simulink model "simulink_test_find_K"  (R2014a)
settings: Solver=ode45  StartTime=0.0  StopTime=5000  RelTol=1e-3
values from neighbouring files (symbols this model uses):
  Gb = 200    [pole_placement.m]    (also in pole_placement2.m; time_domain.m)
  Ib = 0    [pole_placement.m]    (also in pole_placement2.m; time_domain.m)
  n = 0.142    [pole_placement.m]    (also in pole_placement2.m; time_domain.m)
  p1 = 0.035    [pole_placement.m]    (also in pole_placement2.m; time_domain.m)
  p2 = 0.05    [pole_placement.m]    (also in pole_placement2.m; time_domain.m)
  p3 = 0.000023    (= 2.3e-05)    [pole_placement.m]    (also in pole_placement2.m = 2.8e-05; time_domain.m)
  VG = 117    [pole_placement.m]    (also in pole_placement2.m; time_domain.m)
  VI = 1/0.098    (= 10.2040816327)    [pole_placement.m]    (also in pole_placement2.m; time_domain.m)
libraries: simulink x3
settings Model: Creator=joach  LastModifiedBy=joach

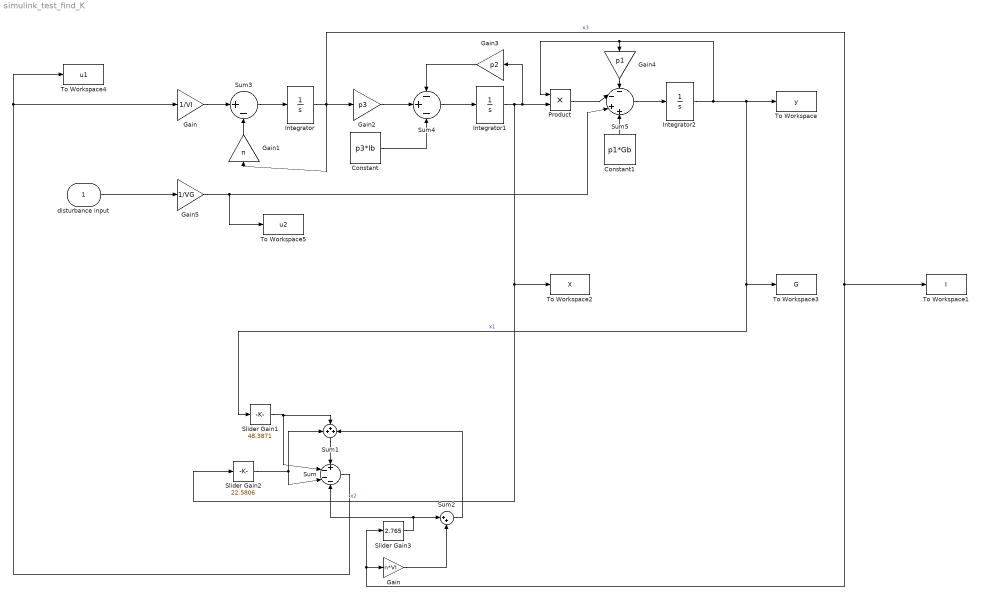
== system simulink_test_find_K ==
  disturbance input : Inport
  " Gain" : Gain  Gain=1/VI
  " Gain2" : Gain  Gain=p3
  " Gain3" : Gain  Gain=p2
  " Gain4" : Gain  Gain=p1
  " Gain5" : Gain  Gain=1/VG
  Constant : Constant  Value=p3*Ib
  Constant1 : Constant  Value=p1*Gb
  Gain : Gain  Gain=n*VI
  Gain1 : Gain  Gain=n
  Integrator : Integrator
  Integrator1 : Integrator
  Integrator2 : Integrator
  Product : Product
  Slider Gain1 : simulink/Math Operations/Slider Gain  low=0  gain=48.3871  high=100
  Slider Gain2 : simulink/Math Operations/Slider Gain  low=0  gain=22.5806  high=100
  Slider Gain3 : simulink/Math Operations/Slider Gain  low=0  gain=2.765  high=100
  Sum : Sum  Inputs=+---
  Sum1 : Sum  Inputs=+++
  Sum2 : Sum  Inputs=|++
  Sum3 : Sum  Inputs=|+-
  Sum4 : Sum  Inputs=-+-
  Sum5 : Sum  Inputs=--++
  To Workspace : ToWorkspace  VariableName=y  SaveFormat=Timeseries  SampleTime=-1
  To Workspace1 : ToWorkspace  VariableName=I  SaveFormat=Timeseries  SampleTime=-1
  To Workspace2 : ToWorkspace  VariableName=X  SaveFormat=Timeseries  SampleTime=-1
  To Workspace3 : ToWorkspace  VariableName=G  SaveFormat=Timeseries  SampleTime=-1
  To Workspace4 : ToWorkspace  VariableName=u1  SaveFormat=Timeseries  SampleTime=-1
  To Workspace5 : ToWorkspace  VariableName=u2  SaveFormat=Timeseries  SampleTime=-1
  wires:
  Sum2/1 -> Sum1/3
  Gain/1 -> Sum2/2
  Slider Gain3/1 -> Sum2/1, Sum/4
  Sum1/1 -> Sum/1
  Slider Gain2/1 -> Sum/3, Sum1/1
  Slider Gain1/1 -> Sum/2, Sum1/2
  Integrator2/1 -> Slider Gain1/1, To Workspace3/1, To Workspace/1, " Gain4"/1, Product/1  "x1"
  Integrator/1 -> To Workspace1/1, Gain/1, Slider Gain3/1, Gain1/1, " Gain2"/1  "x3"
  Integrator1/1 -> " Gain3"/1, Product/2, Slider Gain2/1, To Workspace2/1  "x2"
  Sum/1 -> " Gain"/1, To Workspace4/1
  disturbance input/1 -> " Gain5"/1
  Constant1/1 -> Sum5/4
  " Gain"/1 -> Sum3/1
  Sum5/1 -> Integrator2/1
  Product/1 -> Sum5/2
  " Gain3"/1 -> Sum4/1
  Gain1/1 -> Sum3/2
  Sum4/1 -> Integrator1/1
  " Gain2"/1 -> Sum4/2
  Sum3/1 -> Integrator/1
  Constant/1 -> Sum4/3
  " Gain5"/1 -> To Workspace5/1, Sum5/3
  " Gain4"/1 -> Sum5/1
